simulink model "SWP_IOLinearization"  (R2021a)
settings: Solver=ode1be  StartTime=0.0  StopTime=40  FixedStep=1e-4  RelTol=1e-3
undefined symbols (not defined in the file or in its folder): sigbuilder_block, X, Y, Z
libraries: sm_lib x15, nesl_utility x3
settings Model: Creator=aarti  LastModifiedBy=aarti
settings DataIOCC: ReturnWorkspaceOutputs=off

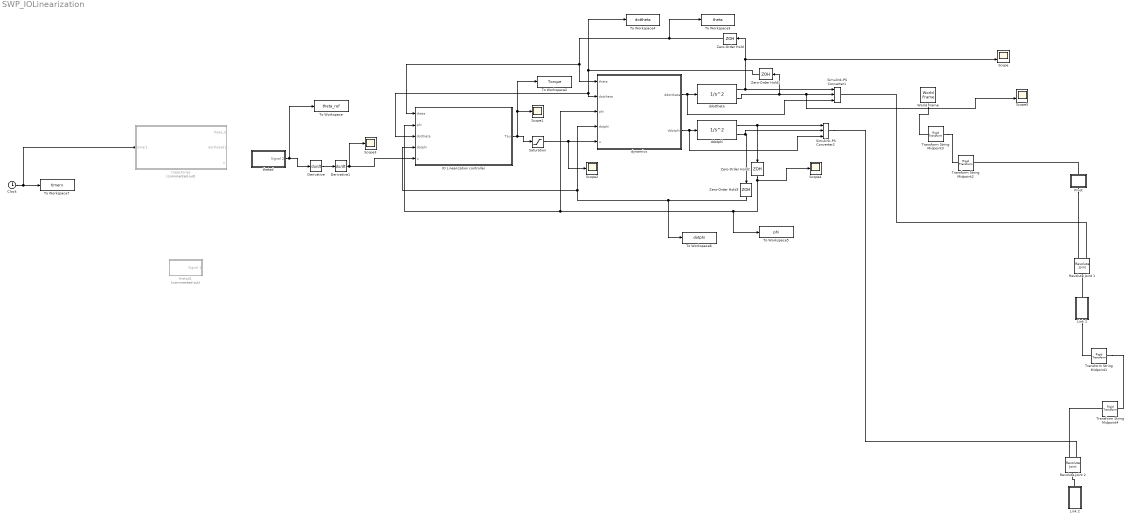
== system SWP_IOLinearization ==
  Clock : Clock
  Derivative : Derivative
  Derivative1 : Derivative
  IO Linearization controller : MATLAB Function  TreatAsAtomicUnit=on
  Link 1 : Subsystem  Tag=CustomStyle
  Link 2 : Subsystem  Tag=CustomStyle
  Pivot : Subsystem  Tag=CustomStyle
  Revolute Joint 1 : sm_lib/Joints/Revolute Joint  JointMode=Normal  SenseConstraintForce=off  SenseConstraintForceX=off  SenseConstraintForceY=off  SenseConstraintForceZ=off  SenseConstraintTorque=off  SenseConstraintTorqueX=off  SenseConstraintTorqueY=off  SenseConstraintTorqueZ=off  SenseTotalForce=off  SenseTotalForceX=off  SenseTotalForceY=off  SenseTotalForceZ=off  SenseTotalTorque=off  SenseTotalTorqueX=off  SenseTotalTorqueY=off  SenseTotalTorqueZ=off  CompositeWrenchDir=FollowerOnBase  CompositeWrenchFrame=BaseFrame  EquilibriumPosition=0  EquilibriumPositionUnits=rad  SpringStiffness=0  SpringStiffnessUnits=N*m/rad  DampingCoefficient=0  DampingCoefficientUnits=N*m/(rad/s)  TorqueActuationMode=ComputedTorque  MotionActuationMode=InputMotion  SensePosition=off  SenseVelocity=off  SenseAcceleration=off  SenseTorqueForce=off  SenseLowerLimitTorqueForce=off  SenseUpperLimitTorqueForce=off  LowerLimitSpecify=off  LowerLimitBound=-90  LowerLimitBoundUnits=deg  LowerLimitStiffness=1e4  LowerLimitStiffnessUnits=N*m/deg  LowerLimitDamping=10  LowerLimitDampingUnits=N*m/(deg/s)  LowerLimitTransitionRegionWidth=0.1  LowerLimitTransitionRegionWidthUnits=deg  UpperLimitSpecify=off  UpperLimitBound=90  UpperLimitBoundUnits=deg  UpperLimitStiffness=1e4  UpperLimitStiffnessUnits=N*m/deg  UpperLimitDamping=10  UpperLimitDampingUnits=N*m/(deg/s)  UpperLimitTransitionRegionWidth=0.1  UpperLimitTransitionRegionWidthUnits=deg  PositionTargetSpecify=off  PositionTargetPriority=High  PositionTargetValue=0  PositionTargetValueUnits=deg  VelocityTargetSpecify=off  VelocityTargetPriority=High  VelocityTargetValue=0  VelocityTargetValueUnits=rad/s
  Revolute Joint 2 : sm_lib/Joints/Revolute Joint  JointMode=Normal  SenseConstraintForce=off  SenseConstraintForceX=off  SenseConstraintForceY=off  SenseConstraintForceZ=off  SenseConstraintTorque=off  SenseConstraintTorqueX=off  SenseConstraintTorqueY=off  SenseConstraintTorqueZ=off  SenseTotalForce=off  SenseTotalForceX=off  SenseTotalForceY=off  SenseTotalForceZ=off  SenseTotalTorque=off  SenseTotalTorqueX=off  SenseTotalTorqueY=off  SenseTotalTorqueZ=off  CompositeWrenchDir=FollowerOnBase  CompositeWrenchFrame=BaseFrame  EquilibriumPosition=0  EquilibriumPositionUnits=rad  SpringStiffness=0  SpringStiffnessUnits=N*m/rad  DampingCoefficient=0  DampingCoefficientUnits=N*m/(rad/s)  TorqueActuationMode=ComputedTorque  MotionActuationMode=InputMotion  SensePosition=off  SenseVelocity=off  SenseAcceleration=off  SenseTorqueForce=off  SenseLowerLimitTorqueForce=off  SenseUpperLimitTorqueForce=off  LowerLimitSpecify=off  LowerLimitBound=-90  LowerLimitBoundUnits=deg  LowerLimitStiffness=1e4  LowerLimitStiffnessUnits=N*m/deg  LowerLimitDamping=10  LowerLimitDampingUnits=N*m/(deg/s)  LowerLimitTransitionRegionWidth=0.1  LowerLimitTransitionRegionWidthUnits=deg  UpperLimitSpecify=off  UpperLimitBound=90  UpperLimitBoundUnits=deg  UpperLimitStiffness=1e4  UpperLimitStiffnessUnits=N*m/deg  UpperLimitDamping=10  UpperLimitDampingUnits=N*m/(deg/s)  UpperLimitTransitionRegionWidth=0.1  UpperLimitTransitionRegionWidthUnits=deg  PositionTargetSpecify=off  PositionTargetPriority=High  PositionTargetValue=0  PositionTargetValueUnits=deg  VelocityTargetSpecify=off  VelocityTargetPriority=High  VelocityTargetValue=0  VelocityTargetValueUnits=rad/s
  Saturation : Saturate  UpperLimit=50  LowerLimit=-50
  Scope : Scope  NumInputPorts=2
  Scope{1..4} (4 alike) : Scope
  Scope5 : Scope  NumInputPorts=2
  Simulink-PS Converter1 : nesl_utility/Simulink-PS Converter  PhysicalDomain=network_engine_domain  SubClassName=ps_input  LeftPortType=input  RightPortType=output  PseudoPeriodic=off  Frequencies=[]  NoiseDistribution=none  NoiseParameters=[]  Unit=1  AffineConversion=off  FilteringAndDerivatives=provide  SimscapeFilterOrder=1  InputFilterTimeConstant=0.001  UdotUserProvided=2
      settings: SourceProductBaseCode=PW,SS
  Simulink-PS Converter2 : nesl_utility/Simulink-PS Converter  PhysicalDomain=network_engine_domain  SubClassName=ps_input  LeftPortType=input  RightPortType=output  PseudoPeriodic=off  Frequencies=[]  NoiseDistribution=none  NoiseParameters=[]  Unit=1  AffineConversion=off  FilteringAndDerivatives=provide  SimscapeFilterOrder=1  InputFilterTimeConstant=0.001  UdotUserProvided=2
      settings: SourceProductBaseCode=PW,SS
  To Workspace : ToWorkspace  VariableName=theta_ref  SampleTime=-1
  To Workspace2 : ToWorkspace  VariableName=Torque  SampleTime=-1
  To Workspace3 : ToWorkspace  VariableName=theta  SampleTime=-1
  To Workspace4 : ToWorkspace  VariableName=dottheta  SampleTime=-1
  To Workspace5 : ToWorkspace  VariableName=phi  SampleTime=-1
  To Workspace6 : ToWorkspace  VariableName=dotphi  SampleTime=-1
  To Workspace7 : ToWorkspace  VariableName=timerx  SampleTime=-1
  Transform String Midpoint1 : sm_lib/Frames and Transforms/Rigid Transform  TranslationMethod=None  TranslationStandardOffset=0  TranslationLengthUnit=m  TranslationStandardAxis=-Y  TranslationCartesianOffset=[0 0 0]  TranslationROffset=0  TranslationROffsetUnits=m  TranslationZOffset=0  TranslationZOffsetUnits=m  TranslationThetaOffset=0  TranslationThetaOffsetUnits=deg  RotationMethod=StandardAxis  RotationAngleUnits=deg  RotationStandardAxis=-X  RotationAngle=90  RotationArbitraryAxis=[0 0 1]  FollAlignAxisA=+X  BaseAlignAxisA=+Y  FollAlignAxisB=+Y  BaseAlignAxisB=+Z  RotationSequenceAxes=FollowerAxes  RotationSequence=XYX  RotationSequenceAngles=[0 0 0]  RotationSequenceAnglesUnits=deg  RotationMatrix=[1 0 0; 0 1 0; 0 0 1]
  Transform String Midpoint2 : sm_lib/Frames and Transforms/Rigid Transform  TranslationMethod=None  TranslationStandardOffset=0  TranslationLengthUnit=m  TranslationStandardAxis=-Y  TranslationCartesianOffset=[0 0 0]  TranslationROffset=0  TranslationROffsetUnits=m  TranslationZOffset=0  TranslationZOffsetUnits=m  TranslationThetaOffset=0  TranslationThetaOffsetUnits=deg  RotationMethod=StandardAxis  RotationAngleUnits=deg  RotationStandardAxis=+X  RotationAngle=90  RotationArbitraryAxis=[0 0 1]  FollAlignAxisA=+X  BaseAlignAxisA=+Y  FollAlignAxisB=+Y  BaseAlignAxisB=+Z  RotationSequenceAxes=FollowerAxes  RotationSequence=XYX  RotationSequenceAngles=[0 0 0]  RotationSequenceAnglesUnits=deg  RotationMatrix=[1 0 0; 0 1 0; 0 0 1]
  Transform String Midpoint3 : sm_lib/Frames and Transforms/Rigid Transform  TranslationMethod=None  TranslationStandardOffset=0  TranslationLengthUnit=m  TranslationStandardAxis=-Y  TranslationCartesianOffset=[0 0 0]  TranslationROffset=0  TranslationROffsetUnits=m  TranslationZOffset=0  TranslationZOffsetUnits=m  TranslationThetaOffset=0  TranslationThetaOffsetUnits=deg  RotationMethod=StandardAxis  RotationAngleUnits=deg  RotationStandardAxis=+Y  RotationAngle=180  RotationArbitraryAxis=[0 0 1]  FollAlignAxisA=+X  BaseAlignAxisA=+Y  FollAlignAxisB=+Y  BaseAlignAxisB=+Z  RotationSequenceAxes=FollowerAxes  RotationSequence=XYX  RotationSequenceAngles=[0 0 0]  RotationSequenceAnglesUnits=deg  RotationMatrix=[1 0 0; 0 1 0; 0 0 1]
  Transform String Midpoint4 : sm_lib/Frames and Transforms/Rigid Transform  TranslationMethod=None  TranslationStandardOffset=0.15/2  TranslationLengthUnit=m  TranslationStandardAxis=-Y  TranslationCartesianOffset=[0 0 0]  TranslationROffset=0  TranslationROffsetUnits=m  TranslationZOffset=0  TranslationZOffsetUnits=m  TranslationThetaOffset=0  TranslationThetaOffsetUnits=deg  RotationMethod=StandardAxis  RotationAngleUnits=deg  RotationStandardAxis=-X  RotationAngle=180  RotationArbitraryAxis=[0 0 1]  FollAlignAxisA=+X  BaseAlignAxisA=+Y  FollAlignAxisB=+Y  BaseAlignAxisB=+Z  RotationSequenceAxes=FollowerAxes  RotationSequence=XYX  RotationSequenceAngles=[0 0 0]  RotationSequenceAnglesUnits=deg  RotationMatrix=[1 0 0; 0 1 0; 0 0 1]
  World Frame : sm_lib/Frames and Transforms/World Frame
  Zero-Order Hold{,1..3} (4 alike) : ZeroOrderHold  SampleTime=-1
  ddotphi : SecondOrderIntegrator  WrapX=on
  ddottheta : SecondOrderIntegrator  WrapX=on
  dynamics : MATLAB Function  TreatAsAtomicUnit=on
  thetad : Subsystem  Tag=STV Subsys  LoadFcn=sigbuilder_block('load');  StartFcn=sigbuilder_block('start');  StopFcn=sigbuilder_block('stop');  ClipboardFcn=sigbuilder_block('clipboard');  mask(Sigbuilder block){tuvar=[0:10]}
      mask help: Simulink:masks:SigbuilderBlock_MD
      mask init:
      | if ~strcmp(get_param(bdroot(gcbh),'SimulationStatus'),'stopped') tuvar = sigbuilder_block('maskInit'); end
      settings: CopyFcn=sigbuilder_block('copy');  DeleteFcn=sigbuilder_block('delete');  ModelCloseFcn=sigbuilder_block('modelClose');  PreSaveFcn=sigbuilder_block('preSave');  PauseFcn=sigbuilder_block('pause');  ContinueFcn=sigbuilder_block('continue');  NameChangeFcn=sigbuilder_block('namechange');  OpenFcn=sigbuilder_block('open',[5.4 5.4 1141.2 580.8 ]);  CloseFcn=sigbuilder_block('close');
      mask Display: plot(0, 0, 100, 100,[2, 2, 32, 32, 2], [68, 8, 8, 68, 68],[32, 2], [38, 38], [32, 19, 2],[53, 60, 44], [32, 17, 17, 2],[16, 16, 31, 31]);txt = getActiveGroup(gcbh);text(2, 100, txt,'verticalAlignment', 'top');
  thetad1 : Subsystem  Tag=STV Subsys  Commented=on  LoadFcn=sigbuilder_block('load');  StartFcn=sigbuilder_block('start');  StopFcn=sigbuilder_block('stop');  ClipboardFcn=sigbuilder_block('clipboard');  mask(Sigbuilder block){tuvar=[0:10]}
      mask help: Simulink:masks:SigbuilderBlock_MD
      mask init:
      | if ~strcmp(get_param(bdroot(gcbh),'SimulationStatus'),'stopped') tuvar = sigbuilder_block('maskInit'); end
      settings: CopyFcn=sigbuilder_block('copy');  DeleteFcn=sigbuilder_block('delete');  ModelCloseFcn=sigbuilder_block('modelClose');  PreSaveFcn=sigbuilder_block('preSave');  PauseFcn=sigbuilder_block('pause');  ContinueFcn=sigbuilder_block('continue');  NameChangeFcn=sigbuilder_block('namechange');  OpenFcn=sigbuilder_block('open',[5.4 36 1141.2 516.6 ]);  CloseFcn=sigbuilder_block('close');
      mask Display: plot(0, 0, 100, 100,[2, 2, 32, 32, 2], [68, 8, 8, 68, 68],[32, 2], [38, 38], [32, 19, 2],[53, 60, 44], [32, 17, 17, 2],[16, 16, 31, 31]);txt = getActiveGroup(gcbh);text(2, 100, txt,'verticalAlignment', 'top');
  trajectories : Subsystem  Commented=on
  wires:
  dynamics/1(ddottheta) -> Simulink-PS Converter1/3, ddottheta/1
  dynamics/2(ddotphi) -> Simulink-PS Converter2/3, ddotphi/1
  ddottheta/1 -> Scope/2, Zero-Order Hold/1, Simulink-PS Converter1/1
  ddottheta/2 -> Zero-Order Hold1/1, Scope5/2, Simulink-PS Converter1/2
  ddotphi/1 -> Simulink-PS Converter2/1, Zero-Order Hold2/1
  ddotphi/2 -> Simulink-PS Converter2/2, Zero-Order Hold3/1
  Zero-Order Hold1/1 -> To Workspace4/1, IO Linearization controller/3(dottheta), dynamics/2(dottheta)
  Zero-Order Hold/1 -> To Workspace3/1, IO Linearization controller/1(theta), dynamics/1(theta)
  Zero-Order Hold2/1 -> Scope4/1, To Workspace5/1, dynamics/3(phi), IO Linearization controller/2(phi)
  Zero-Order Hold3/1 -> To Workspace6/1, dynamics/4(dotphi), IO Linearization controller/4(dotphi)
  Clock/1 -> trajectories/1(timer1), To Workspace7/1
  IO Linearization controller/1(Tau) -> Saturation/1, To Workspace2/1, Scope1/1
  Saturation/1 -> Scope2/1, dynamics/5(u)
  thetad/1(Signal 2) -> To Workspace/1, Derivative/1
  Derivative/1 -> Derivative1/1
  Derivative1/1 -> Scope3/1, IO Linearization controller/5(u)
  connections:
  Link 2/RConn1 -- Revolute Joint 2/RConn1
  Pivot/LConn1 -- Transform String Midpoint2/LConn1
  Transform String Midpoint3/LConn1 -- Transform String Midpoint2/RConn1
  Pivot/RConn1 -- Revolute Joint 1/LConn1
  Simulink-PS Converter2/RConn1 -- Revolute Joint 2/LConn2
  Revolute Joint 1/LConn2 -- Simulink-PS Converter1/RConn1
  Transform String Midpoint1/LConn1 -- Transform String Midpoint4/LConn1
  Link 1/LConn1 -- Transform String Midpoint1/RConn1
  Link 1/RConn1 -- Revolute Joint 1/RConn1
  Transform String Midpoint4/RConn1 -- Revolute Joint 2/LConn1
  World Frame/RConn1 -- Transform String Midpoint3/RConn1

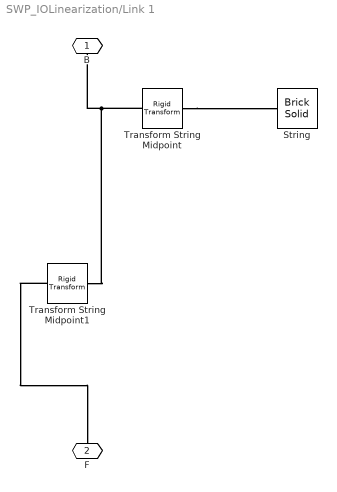
== system SWP_IOLinearization/Link 1 ==
  String : sm_lib/Body Elements/Brick Solid  GraphicAmbientColor=[0.15 0.15 0.15 1.0]  BasedOnType=Density  BrickDimensions=[0.012 0.25 0.012]  BrickDimensionUnits=m  CenterOfMass=[0 0 0]  CenterOfMassUnits=m  GraphicDiffuseColor=[0.3764706 0.21568628 0.3764706]  Density=0  DensityUnits=kg/(m^3)  DoExposeReferenceFrame=on  GraphicEmissiveColor=[0.0 0.0 0.0 1.0]  ExportEntireGeometry=off  SerializedFrames=<Frames/>  MarkerShape=Sphere  MarkerSize=10  GraphicType=FromGeometry  InertiaType=PointMass  Mass=0  MassUnits=kg  MomentsOfInertia=[1 1 1]*1e-3  MomentsOfInertiaUnits=kg*m^2  GraphicOpacity=1.0  ProductsOfInertia=[0 0 0]  ProductsOfInertiaUnits=kg*m^2  GraphicShininess=75  GraphicSpecularColor=[0.5 0.5 0.5 1.0]  GraphicVisPropType=SimpleVisualProperties
  Transform String Midpoint : sm_lib/Frames and Transforms/Rigid Transform  TranslationMethod=StandardAxis  TranslationStandardOffset=0.25/2  TranslationLengthUnit=m  TranslationStandardAxis=-Y  TranslationCartesianOffset=[0 0 0]  TranslationROffset=0  TranslationROffsetUnits=m  TranslationZOffset=0  TranslationZOffsetUnits=m  TranslationThetaOffset=0  TranslationThetaOffsetUnits=deg  RotationMethod=None  RotationAngleUnits=deg  RotationStandardAxis=+Z  RotationAngle=0  RotationArbitraryAxis=[0 0 1]  FollAlignAxisA=+X  BaseAlignAxisA=+Y  FollAlignAxisB=+Y  BaseAlignAxisB=+Z  RotationSequenceAxes=FollowerAxes  RotationSequence=XYX  RotationSequenceAngles=[0 0 0]  RotationSequenceAnglesUnits=deg  RotationMatrix=[1 0 0; 0 1 0; 0 0 1]
  Transform String Midpoint1 : sm_lib/Frames and Transforms/Rigid Transform  TranslationMethod=StandardAxis  TranslationStandardOffset=0.25  TranslationLengthUnit=m  TranslationStandardAxis=-Y  TranslationCartesianOffset=[0 0 0]  TranslationROffset=0  TranslationROffsetUnits=m  TranslationZOffset=0  TranslationZOffsetUnits=m  TranslationThetaOffset=0  TranslationThetaOffsetUnits=deg  RotationMethod=None  RotationAngleUnits=deg  RotationStandardAxis=+Z  RotationAngle=0  RotationArbitraryAxis=[0 0 1]  FollAlignAxisA=+X  BaseAlignAxisA=+Y  FollAlignAxisB=+Y  BaseAlignAxisB=+Z  RotationSequenceAxes=FollowerAxes  RotationSequence=XYX  RotationSequenceAngles=[0 0 0]  RotationSequenceAnglesUnits=deg  RotationMatrix=[1 0 0; 0 1 0; 0 0 1]
  B : PMIOPort  Side=Right
  F : PMIOPort  Port=2  Side=Left
  connections:
  Transform String Midpoint/RConn1 -- String/RConn1
  Transform String Midpoint/LConn1 -- Transform String Midpoint1/LConn1 -- B/RConn1
  Transform String Midpoint1/RConn1 -- F/RConn1

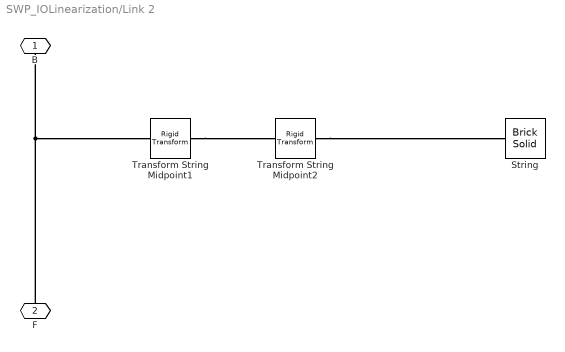
== system SWP_IOLinearization/Link 2 ==
  String : sm_lib/Body Elements/Brick Solid  GraphicAmbientColor=[0.15 0.15 0.15 1.0]  BasedOnType=Density  BrickDimensions=[0.015 0.15 0.015]  BrickDimensionUnits=m  CenterOfMass=[0 0 0]  CenterOfMassUnits=m  GraphicDiffuseColor=[0.011764706 0.40392157 0.6392157]  Density=0  DensityUnits=kg/(m^3)  DoExposeReferenceFrame=on  GraphicEmissiveColor=[0.0 0.0 0.0 1.0]  ExportEntireGeometry=off  SerializedFrames=<Frames/>  MarkerShape=Sphere  MarkerSize=10  GraphicType=FromGeometry  InertiaType=PointMass  Mass=0  MassUnits=kg  MomentsOfInertia=[1 1 1]*1e-3  MomentsOfInertiaUnits=kg*m^2  GraphicOpacity=1.0  ProductsOfInertia=[0 0 0]  ProductsOfInertiaUnits=kg*m^2  GraphicShininess=75  GraphicSpecularColor=[0.5 0.5 0.5 1.0]  GraphicVisPropType=SimpleVisualProperties
  Transform String Midpoint1 : sm_lib/Frames and Transforms/Rigid Transform  TranslationMethod=StandardAxis  TranslationStandardOffset=0.15/2  TranslationLengthUnit=m  TranslationStandardAxis=-Y  TranslationCartesianOffset=[0 0 0]  TranslationROffset=0  TranslationROffsetUnits=m  TranslationZOffset=0  TranslationZOffsetUnits=m  TranslationThetaOffset=0  TranslationThetaOffsetUnits=deg  RotationMethod=StandardAxis  RotationAngleUnits=deg  RotationStandardAxis=-Z  RotationAngle=180  RotationArbitraryAxis=[0 0 1]  FollAlignAxisA=+X  BaseAlignAxisA=+Y  FollAlignAxisB=+Y  BaseAlignAxisB=+Z  RotationSequenceAxes=FollowerAxes  RotationSequence=XYX  RotationSequenceAngles=[0 0 0]  RotationSequenceAnglesUnits=deg  RotationMatrix=[1 0 0; 0 1 0; 0 0 1]
  Transform String Midpoint2 : sm_lib/Frames and Transforms/Rigid Transform  TranslationMethod=None  TranslationStandardOffset=0.15/2  TranslationLengthUnit=m  TranslationStandardAxis=-Y  TranslationCartesianOffset=[0 0 0]  TranslationROffset=0  TranslationROffsetUnits=m  TranslationZOffset=0  TranslationZOffsetUnits=m  TranslationThetaOffset=0  TranslationThetaOffsetUnits=deg  RotationMethod=StandardAxis  RotationAngleUnits=deg  RotationStandardAxis=+X  RotationAngle=0  RotationArbitraryAxis=[0 0 1]  FollAlignAxisA=+X  BaseAlignAxisA=+Y  FollAlignAxisB=+Y  BaseAlignAxisB=+Z  RotationSequenceAxes=FollowerAxes  RotationSequence=XYX  RotationSequenceAngles=[0 0 0]  RotationSequenceAnglesUnits=deg  RotationMatrix=[1 0 0; 0 1 0; 0 0 1]
  B : PMIOPort  Side=Right
  F : PMIOPort  Port=2  Side=Left
  connections:
  Transform String Midpoint1/LConn1 -- Transform String Midpoint2/RConn1
  F/RConn1 -- Transform String Midpoint1/RConn1 -- B/RConn1
  Transform String Midpoint2/LConn1 -- String/RConn1

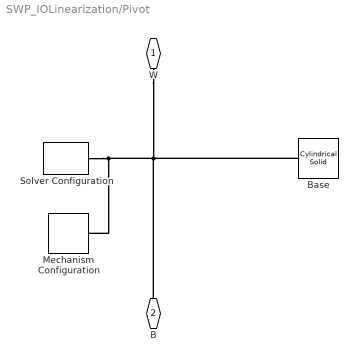
== system SWP_IOLinearization/Pivot ==
  Base : sm_lib/Body Elements/Cylindrical Solid  GraphicAmbientColor=[0.15 0.15 0.15 1.0]  BasedOnType=Density  CenterOfMass=[0 0 0]  CenterOfMassUnits=m  GraphicDiffuseColor=[0.3 0.3 0.3]  CylinderLength=0.4  CylinderLengthUnits=m  CylinderRadius=0.01  CylinderRadiusUnits=m  Density=1000  DensityUnits=kg/(m^3)  DoExposeReferenceFrame=on  GraphicEmissiveColor=[0.0 0.0 0.0 1.0]  ExportEntireGeometry=off  SerializedFrames=<Frames/>  MarkerShape=Sphere  MarkerSize=10  GraphicType=FromGeometry  InertiaType=PointMass  Mass=10  MassUnits=kg  MomentsOfInertia=[1 1 1]*1e-3  MomentsOfInertiaUnits=kg*m^2  GraphicOpacity=1.0  ProductsOfInertia=[0 0 0]  ProductsOfInertiaUnits=kg*m^2  GraphicShininess=75  GraphicSpecularColor=[0.5 0.5 0.5 1.0]  GraphicVisPropType=AdvancedVisualProperties
  Mechanism Configuration : sm_lib/Utilities/Mechanism Configuration  UniformGravity=Constant  GravityVector=[0 0 -9.81]  GravityVectorUnits=m/s^2  GravityUnits=m/s^2  LinearizationDelta=0.001  JointModeTransitionNonlinearIterations=2
  Solver Configuration : nesl_utility/Solver Configuration  PhysicalDomain=network_engine_domain  SubClassName=solver  LeftPortType=input  RightPortType=generic  Tones=[]  Harmonics=[]  SimulateNoise=off  Profile=off  UseLocalSampling=off  EnableSwitchedLinearOptims=on  FrequencyDomain=off  UseCCode=off  RelTol=0.001  AbsTol=1e-06  MinStep=1e-09  ToWorkspace=off  RevertToSquareIcSolve=off  NumHomotopyIterations=100  PhasorMode=off  PhasorModeNumHarmonics=1  DoDC=on  ResidualTolerance=1e-9  UseLocalSolver=off  LocalSolverChoice=NE_BACKWARD_EULER_ADVANCER  LocalSolverSampleTime=.001  DoFixedCost=off  MaxNonlinIter=3  MaxModeIter=2  ComputeImpulses=off  ImpulseIterations=2  LinearAlgebra=Sparse  EquationFormulation=NE_TIME_EF  DelaysMemoryBudget=1024  AutomaticFiltering=on  FilteringTimeConstant=0.001  PartitionStorageMethod=AS_NEEDED  PartitionMemoryBudget=1024  PartitionMethod=FAST
      settings: SourceProductBaseCode=PW,SS
  W : PMIOPort  Side=Left
  B : PMIOPort  Port=2  Side=Right
  connections:
  W/RConn1 -- B/RConn1 -- Base/RConn1 -- Solver Configuration/RConn1 -- Mechanism Configuration/RConn1

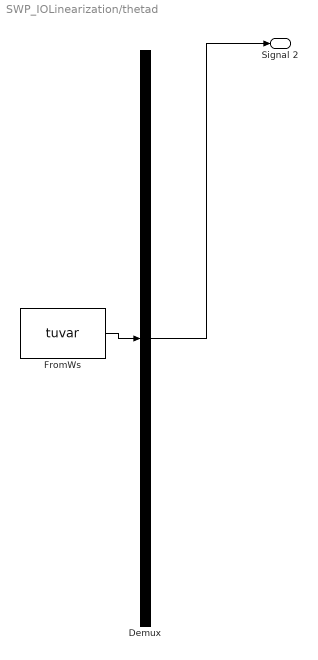
== system SWP_IOLinearization/thetad ==
  Demux : Demux  Tag=STV Demux  Outputs=1
      settings: DisplayOption=none
  FromWs : FromWorkspace  Tag=STV FromWs  VariableName=tuvar
      SigBuilderData=|
      | common.afterFinalStr = 'Extrapolate'
      | common.sampleTime = 0
      | dataSet.timeRange = [0 40]
      | dataSet.name = 'Group 1'
      | sbobj.Groups.Name = 'Group 1'
      | sbobj.Groups.Signals.Name = 'Signal 2'
      | sbobj.Groups.Signals.XData = [0 0.0408163265306 0.0816326530612 0.122448979592 0.163265306122 0.204081632653 0.244897959184 0.285714285714 0.326530612245 0.367346938776 0.408163265306 0.448979591837 ... (249 elements, 1x249)]
      | sbobj.Groups.Signals.YData = [0 0.0383631485054 0.0760963751729 0.112580101464 0.147215265601 0.179433159147 0.208704765181 0.23454944474 0.256542828902 0.274323786905 0.287600355911 0.296154535024 ... (249 elements, 1x249)]
      | sbobj.Groups.TimeRange = [0 40]
  Signal 2 : Outport  Tag=STV Outport
  wires:
  FromWs/1 -> Demux/1
  Demux/1 -> Signal 2/1

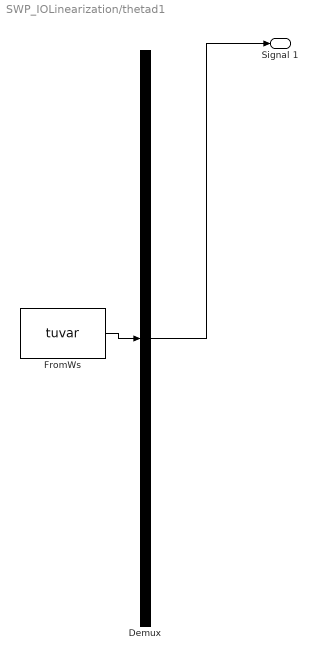
== system SWP_IOLinearization/thetad1 ==
  Demux : Demux  Tag=STV Demux  Outputs=1
      settings: DisplayOption=none
  FromWs : FromWorkspace  Tag=STV FromWs  VariableName=tuvar
      SigBuilderData=|
      | common.afterFinalStr = 'Extrapolate'
      | common.sampleTime = 0
      | dataSet.timeRange = [0 40]
      | dataSet.name = 'Group 1'
      | sbobj.Groups.Name = 'Group 1'
      | sbobj.Groups.Signals.Name = 'Signal 1'
      | sbobj.Groups.Signals.XData = [0 0.0408163265306 0.0816326530612 0.122448979592 0.163265306122 0.204081632653 0.244897959184 0.285714285714 0.326530612245 0.367346938776 0.408163265306 0.448979591837 ... (249 elements, 1x249)]
      | sbobj.Groups.Signals.YData = [0 0.0153452594021 0.0304385500691 0.0450320405855 0.0588861062405 0.0717732636589 0.0834819060724 0.0938197778962 0.102617131561 0.109729514762 0.115040142364 0.11846181401 ... (249 elements, 1x249)]
      | sbobj.Groups.TimeRange = [0 40]
  Signal 1 : Outport  Tag=STV Outport
  wires:
  FromWs/1 -> Demux/1
  Demux/1 -> Signal 1/1

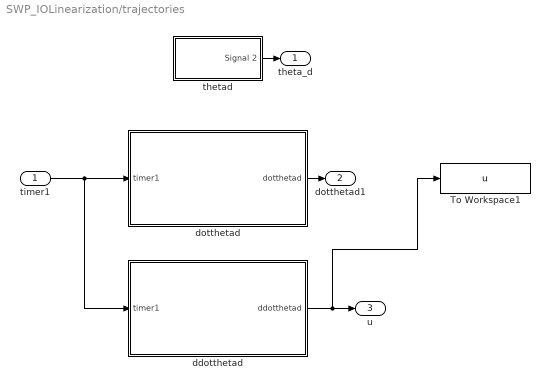
== system SWP_IOLinearization/trajectories ==
  timer1 : Inport
  To Workspace1 : ToWorkspace  VariableName=u  SampleTime=-1
  ddotthetad : MATLAB Function  TreatAsAtomicUnit=on
  dotthetad : MATLAB Function  TreatAsAtomicUnit=on
  thetad : Subsystem  Tag=STV Subsys  LoadFcn=sigbuilder_block('load');  StartFcn=sigbuilder_block('start');  StopFcn=sigbuilder_block('stop');  ClipboardFcn=sigbuilder_block('clipboard');  mask(Sigbuilder block){tuvar=[0:10]}
      mask help: Simulink:masks:SigbuilderBlock_MD
      mask init:
      | if ~strcmp(get_param(bdroot(gcbh),'SimulationStatus'),'stopped') tuvar = sigbuilder_block('maskInit'); end
      settings: CopyFcn=sigbuilder_block('copy');  DeleteFcn=sigbuilder_block('delete');  ModelCloseFcn=sigbuilder_block('modelClose');  PreSaveFcn=sigbuilder_block('preSave');  PauseFcn=sigbuilder_block('pause');  ContinueFcn=sigbuilder_block('continue');  NameChangeFcn=sigbuilder_block('namechange');  OpenFcn=sigbuilder_block('open',[5.4 5.4 1141.2 580.8 ]);  CloseFcn=sigbuilder_block('close');
      mask Display: plot(0, 0, 100, 100,[2, 2, 32, 32, 2], [68, 8, 8, 68, 68],[32, 2], [38, 38], [32, 19, 2],[53, 60, 44], [32, 17, 17, 2],[16, 16, 31, 31]);txt = getActiveGroup(gcbh);text(2, 100, txt,'verticalAlignment', 'top');
  theta_d : Outport
  dotthetad1 : Outport  Port=2
  u : Outport  Port=3
  wires:
  ddotthetad/1(ddotthetad) -> To Workspace1/1, u/1
  dotthetad/1(dotthetad) -> dotthetad1/1
  thetad/1(Signal 2) -> theta_d/1
  timer1/1 -> ddotthetad/1(timer1), dotthetad/1(timer1)

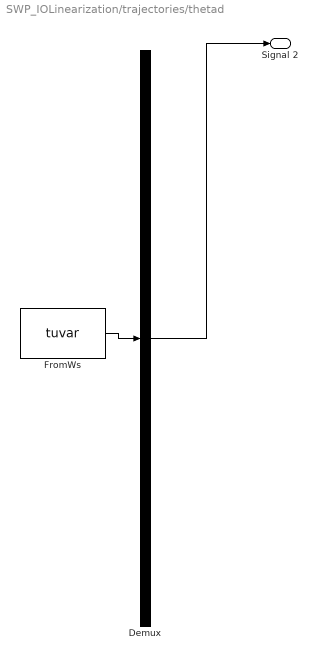
== system SWP_IOLinearization/trajectories/thetad ==
  Demux : Demux  Tag=STV Demux  Outputs=1
      settings: DisplayOption=none
  FromWs : FromWorkspace  Tag=STV FromWs  VariableName=tuvar
      SigBuilderData=|
      | common.afterFinalStr = 'Extrapolate'
      | common.sampleTime = 0
      | dataSet.timeRange = [0 40]
      | dataSet.name = 'Group 1'
      | sbobj.Groups.Name = 'Group 1'
      | sbobj.Groups.Signals.Name = 'Signal 2'
      | sbobj.Groups.Signals.XData = [0 0.0408163265306 0.0816326530612 0.122448979592 0.163265306122 0.204081632653 0.244897959184 0.285714285714 0.326530612245 0.367346938776 0.408163265306 0.448979591837 ... (249 elements, 1x249)]
      | sbobj.Groups.Signals.YData = [0 0.0383631485054 0.0760963751729 0.112580101464 0.147215265601 0.179433159147 0.208704765181 0.23454944474 0.256542828902 0.274323786905 0.287600355911 0.296154535024 ... (249 elements, 1x249)]
      | sbobj.Groups.TimeRange = [0 40]
  Signal 2 : Outport  Tag=STV Outport
  wires:
  FromWs/1 -> Demux/1
  Demux/1 -> Signal 2/1

== matlab function SWP_IOLinearization/dynamics ==
  data: theta input; ddottheta output; dottheta input; phi input; dotphi input; u input; ddotphi output
function [ddottheta,ddotphi]=SwirlingPendulum(theta,dottheta,phi,dotphi,u)
%% Swirling Pendulum Equations of Motion
%Define the parameter values
% m1 = 0.465;
% m2 = 0.085;
% l1 = 0.13;
% l2 = 0.145 ;
m1 = 0.435 ;
m2 = 0.325 ;
l1 = 0.07 ;
l2 = 0.0855 ;
g = 9.81;
% m1 = 0.01353; 
% m2 = 0.209; 
% l1 =0.093; 
% l2 =0.114;
% b1 = 0.002 ;
% % b2 = 0.002 ;
% g = 9.81; 
% Inertia Matrix
    M=[4/3*(m1*l1^2+m2*(3*l1^2+(l2*sin(phi))^2)), 2*m2*l1*l2*cos(phi);
    2*m2*l1*l2*cos(phi), 4/3*(m2*l2^2)];
% Coriolis 
    C = [(4/3)*m2*l2*l2*sin(phi)*cos(phi)*dotphi, (4/3)*m2*l2*l2*sin(phi)*cos(phi)*dottheta - 2*m2*l1*l2*sin(phi)*dotphi;
    (-4/3)*m2*l2*l2*cos(phi)*sin(phi)*dottheta, 0];
% Potential Terms
    G=[(m1+2*m2)*g*l1*sin(theta)+m2*g*l2*sin(phi)*cos(theta);m2*g*l2*sin(theta)*cos(phi)];
% % Viscous friction
%     D = [b1*dottheta;b2*dotphi] ;
%Mx''+Cx'+G+D = Bu;
B = [0;1] ;
ddotX=inv(M)*(-C*[dottheta;dotphi]-G+B*u);
ddottheta=ddotX(1,:);
ddotphi=ddotX(2,:);

== matlab function SWP_IOLinearization/IO Linearization controller ==
  data: Tau output; theta input; phi input; dottheta input; dotphi input; u input
function Tau = fcn(theta,phi,dottheta,dotphi,u)
% m1 = 0.465 ;
% m2 = 0.085 ;
% l1 = 0.13 ;
% l2 = 0.145 ;
m1 = 0.435 ;
m2 = 0.325 ;
l1 = 0.07 ;
l2 = 0.0855 ;
g = 9.81 ;
siga = 2*(4*m1*l1^2*l2 + 12*m2*l1^2*l2 + 4*m2*l2^3*(sin(phi))^2 - 9*m2*l1^2 ...
    *l2*(cos(phi))^2) ;
sigb = (8*m1*l1^2 + 24*m2*l1^2 + 8*m2*l2^2 - 18*m2*l1^2*(cos(phi))^2 - ...
    8*m2*l2^2*(cos(phi))^2)*u + 6*g*m1*l1*sin(theta) + 12*m2*g*l1*sin(theta) ...
    - 12*m2*l1*l2*dotphi^2*sin(phi) + 6*m2*g*l2*cos(theta)*sin(phi) - ...
    9*m2*g*l1*(cos(phi))^2*sin(theta) + 16*m2*l2^2*dotphi*dottheta*cos(phi) ...
    *sin(phi) + 12*m2*l1*l2*dottheta^2*sin(phi)*(cos(phi))^2 ;
sigc = 9*l1*cos(phi)*(8*m1*l1^2 + 24*m2*l1^2 + 8*m2*l2^2 - 18*m2*l1^2* ...
    (cos(phi))^2 - 8*m2*l2^2*(cos(phi))^2) ;
Tau = -(siga*sigb)/sigc ;
end

== matlab function SWP_IOLinearization/trajectories/dotthetad ==
  data: timer1 input; dotthetad output
function dotthetad = fcn(timer1)
    amp = 0.3 ; w = pi ;   
    if(timer1 < 10)
      dotthetad = amp*w*cos(w*timer1) ;    
    elseif(timer1>10 || timer1 < 10)
      dotthetad = 0.03 ;
    elseif(timer1>20 || timer1<30)
      dotthetad = 0 ;
    else
      dotthetad = - 0.03 ;  
    end    
end

== matlab function SWP_IOLinearization/trajectories/ddotthetad ==
  data: timer1 input; ddotthetad output
function ddotthetad = fcn(timer1)
    amp = 0.3 ; w = pi ;   
    if(timer1 < 10)
      ddotthetad = -amp*w^2*sin(w*timer1) ;    
    elseif(timer1>10 || timer1 < 10)
      ddotthetad = 0 ;
    elseif(timer1>20 || timer1<30)
      ddotthetad = 0 ;
    else
      ddotthetad = 0 ;  
    end    
end
